simulink model "Lock_In"  (Simulink 4.00)
settings: Solver=ode45  StartTime=0.0  StopTime=1  RelTol=1e-5
libraries: dsparch3 x2
settings Model: LastModifiedBy=pdrljaca  BlockReductionOpt=off

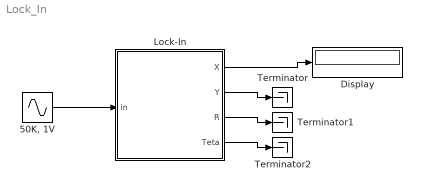
== system Lock_In ==
  "50K, 1V" : Sin  Amplitude=1  Frequency=50000  Phase=0  SampleTime=0
  Display : Display
      settings: Format=short  SampleTime=0.1
  Lock-In : Subsystem  Description=Lock in Amplifier  mask{freq=50000, harmonic=1, order=1, pass=10}
      mask prompts: freq "Detection frequency (rad/sec)"; order "FilterOrder"; pass "Pass band edge frequency"
      mask help:
      | LOCK-IN AMPLIFIER
      | Copyright (c) Predrag Drljaca 2002
      | Choose internal frequency of the clock generator, harminic of the signal you want to measure, as well as the order and the frequency of the internal low pass filter.
      settings: RTWFcnNameOpts=Auto  RTWFileNameOpts=Auto
      mask Display:
      | plot([1 40 40 60 60 90], [3 3 50 50 3 3]);
      | text(7,60,'Lock-in ampli');
      | plot([0 1], [65 65]);
  Terminator : Terminator
  Terminator1 : Terminator
  Terminator2 : Terminator
  wires:
  Lock-In/4(Teta) -> Terminator2/1
  Lock-In/3(R) -> Terminator1/1
  Lock-In/2(Y) -> Terminator/1
  "50K, 1V"/1 -> Lock-In/1(in)
  Lock-In/1(X) -> Display/1

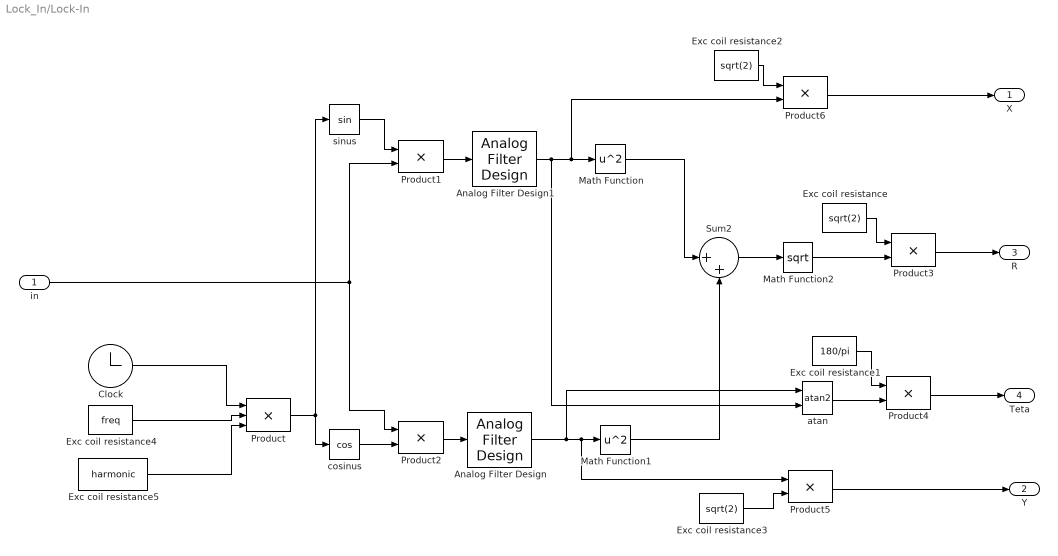
== system Lock_In/Lock-In ==
  in : Inport  Port=1
  Analog Filter Design : dsparch3/Analog Filter Design  method=Butterworth  filttype=Lowpass  N=order  Wlo=pass  Whi=80  Rp=2  Rs=40
  Analog Filter Design1 : dsparch3/Analog Filter Design  method=Butterworth  filttype=Lowpass  N=order  Wlo=pass  Whi=80  Rp=2  Rs=40
  Clock : Clock
      settings: DisplayTime=off  Decimation=10
  Exc coil resistance : Constant  Value=sqrt(2)
  Exc coil resistance1 : Constant  Value=180/pi
  Exc coil resistance2 : Constant  Value=sqrt(2)
  Exc coil resistance3 : Constant  Value=sqrt(2)
  Exc coil resistance4 : Constant  Value=freq
  Exc coil resistance5 : Constant  Value=harmonic
  Math Function : Math  Operator=square  OutputSignalType=auto
  Math Function1 : Math  Operator=square  OutputSignalType=auto
  Math Function2 : Math  Operator=sqrt  OutputSignalType=auto
  Product : Product  Inputs=***  Multiplication=Element-wise(.*)  SaturateOnIntegerOverflow=on
  Product{1..6} (6 alike) : Product  Inputs=2  Multiplication=Element-wise(.*)  SaturateOnIntegerOverflow=on
  Sum2 : Sum  Inputs=|++  SaturateOnIntegerOverflow=on
  atan : Trigonometry  Operator=atan2  OutputSignalType=real
  cosinus : Trigonometry  Operator=cos  OutputSignalType=auto
  sinus : Trigonometry  Operator=sin  OutputSignalType=auto
  X : Outport  Port=1
  Y : Outport  Port=2
  R : Outport  Port=3
  Teta : Outport  Port=4
  wires:
  Product5/1 -> Y/1
  Product1/1 -> Analog Filter Design1/1
  Product2/1 -> Analog Filter Design/1
  Exc coil resistance2/1 -> Product6/1
  Product6/1 -> X/1
  Exc coil resistance3/1 -> Product5/2
  Math Function1/1 -> Sum2/2
  Analog Filter Design/1 -> Product5/1, Math Function1/1, atan/1
  Math Function/1 -> Sum2/1
  Analog Filter Design1/1 -> Product6/2, Math Function/1, atan/2
  Exc coil resistance1/1 -> Product4/1
  Product4/1 -> Teta/1
  atan/1 -> Product4/2
  Exc coil resistance/1 -> Product3/1
  Product3/1 -> R/1
  Math Function2/1 -> Product3/2
  Sum2/1 -> Math Function2/1
  cosinus/1 -> Product2/2
  in/1 -> Product2/1, Product1/2
  sinus/1 -> Product1/1
  Exc coil resistance4/1 -> Product/2
  Product/1 -> sinus/1, cosinus/1
  Clock/1 -> Product/1
  Exc coil resistance5/1 -> Product/3
